simulink model "ACT_ATT"  (R2020a)
settings: Solver=VariableStepAuto  StartTime=0.0  StopTime=10.0  RelTol=1e-3
settings Model: Creator=m_mam  LastModifiedBy=m_mam

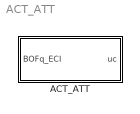
== system ACT_ATT ==
  ACT_ATT : Subsystem

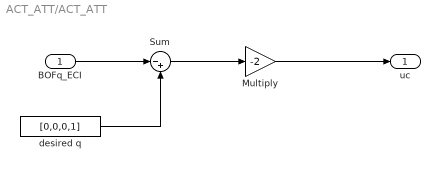
== system ACT_ATT/ACT_ATT ==
  BOFq_ECI : Inport
  Multiply : Gain  Gain=-2
  Sum : Sum  Inputs=|-+
  desired q : Constant  Value=[0,0,0,1]
  uc : Outport
  wires:
  desired q/1 -> Sum/2
  BOFq_ECI/1 -> Sum/1
  Sum/1 -> Multiply/1
  Multiply/1 -> uc/1
